simulink model "untitled"  (R2023a)
settings: Solver=VariableStepAuto  StartTime=0.0  StopTime=1  RelTol=1e-3
settings Model: Creator=Anikait  LastModifiedBy=Anikait

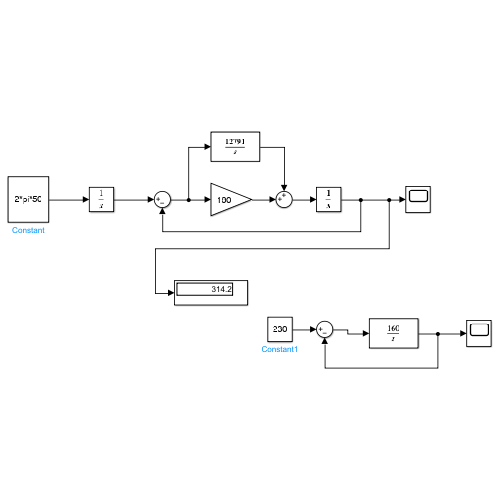
[thumbnail: Simulink's stored preview of the top-level diagram]
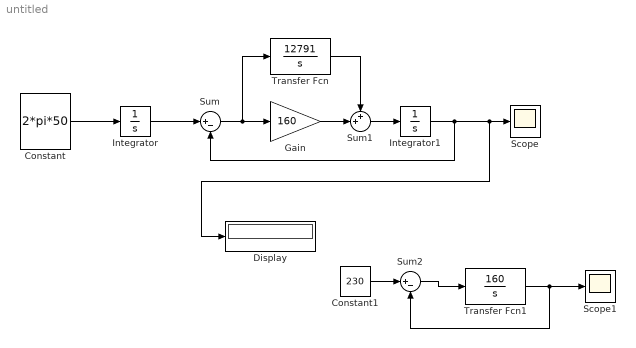
== system untitled ==
  Constant : Constant  Value=2*pi*50
  Constant1 : Constant  Value=230
  Display : Display
  Gain : Gain  Gain=160
  Integrator : Integrator
  Integrator1 : Integrator
  Scope : Scope
  Scope1 : Scope
  Sum : Sum  Inputs=|+-
  Sum1 : Sum  Inputs=++|
  Sum2 : Sum  Inputs=|+-
  Transfer Fcn : TransferFcn  Numerator=[12791]  Denominator=[1 0]
  Transfer Fcn1 : TransferFcn  Numerator=[160]  Denominator=[1 0]
  wires:
  Sum/1 -> Transfer Fcn/1, Gain/1
  Gain/1 -> Sum1/2
  Transfer Fcn/1 -> Sum1/1
  Sum1/1 -> Integrator1/1
  Integrator1/1 -> Sum/2, Display/1, Scope/1
  Constant/1 -> Integrator/1
  Sum2/1 -> Transfer Fcn1/1
  Transfer Fcn1/1 -> Scope1/1, Sum2/2
  Constant1/1 -> Sum2/1
  Integrator/1 -> Sum/1
